simulink model "Seven_dof2017a"  (R2017a)
settings: Solver=ode45  StartTime=0.0  StopTime=10.0  RelTol=1e-3
values from neighbouring files (symbols this model uses):
  Bf = 1.6    [0108.mat]    (also in Sensor_wz_u1.m; Sensor_wz_u3.m; Sensor_wz_u4.m; unlinear_7DOF_Parameters.m)
  Br = 1.6    [0108.mat]    (also in Sensor_wz_u1.m; Sensor_wz_u3.m; Sensor_wz_u4.m; unlinear_7DOF_Parameters.m)
  f = 0.015    [0108.mat]    (also in unlinear_7DOF_Parameters.m)
  g = 9.8    [0108.mat]    (also in unlinear_7DOF_Parameters.m)
  hg = 0.5    [0108.mat]    (also in unlinear_7DOF_Parameters.m)
  i_sw = 20    [unlinear_7DOF_Parameters.m]
  I_tire = 2.5    [0108.mat]    (also in unlinear_7DOF_Parameters.m)
  Iz = 2700    [0108.mat]    (also in LinearState2_u.m = 1536.7; Sensor_wz_u1.m; Sensor_wz_u3.m; Sensor_wz_u4.m)
  L = 2.6    [0108.mat]    (also in unlinear_7DOF_Parameters.m)
  Lf = 1.2    [0108.mat]    (also in Sensor_wz_u1.m; Sensor_wz_u3.m; Sensor_wz_u4.m; unlinear_7DOF_Parameters.m)
  Lr = 1.4    [0108.mat]    (also in Sensor_wz_u1.m = 1.2; Sensor_wz_u3.m = 1.2; Sensor_wz_u4.m = 1.2; unlinear_7DOF_Parameters.m)
  m = 1765    [0108.mat]    (also in LinearState2_u.m = 1412; Sensor_ax_u0.m; Sensor_ax_u1.m; Sensor_ax_u2.m = 1412)
  mb = 1600    [0108.mat]    (also in unlinear_7DOF_Parameters.m)
  mw = 41.25    [0108.mat]    (also in unlinear_7DOF_Parameters.m)
  Pn_motor = 80    [unlinear_7DOF_Parameters.m]
  r = 0.324956275    [0108.mat]    (also in unlinear_7DOF_Parameters.m = 0.354)
  Tn_motor = 1000    [unlinear_7DOF_Parameters.m]
  u_fl = 0.3    [unlinear_7DOF_Parameters.m]
  u_fr = 0.8    [unlinear_7DOF_Parameters.m]
  u_rl = 0.3    [unlinear_7DOF_Parameters.m]
  u_rr = 0.8    [unlinear_7DOF_Parameters.m]
  v_obj = 16    [unlinear_7DOF_Parameters.m]
  vx0 = 16    [unlinear_7DOF_Parameters.m]
  w0 = vx0/r    (= 45.197740113)    [unlinear_7DOF_Parameters.m]
libraries: sharedTrackingLibrary x2, simulink x1
(part 1 of 2)
settings Model: Creator=dzY  LastModifiedBy=dzY
settings DataIOCC: LimitDataPoints=on  SaveFormat=Array
settings OptimizationCC: BlockReduction=off  BooleanDataType=off  LifeSpan=inf
settings DebuggingCC: SaveWithParameterizedLinksMsg=none  UnderspecifiedInitializationDetection=Classic  MergeDetectMultiDrivingBlocksExec=none  SignalResolutionControl=TryResolveAllWithWarning  SFUnexpectedBacktrackingDiag=warning  SFNoUnconditionalDefaultTransitionDiag=warning  SFExecutionAtInitializationDiag=none
settings HardwareCC: ProdBitPerPointer=32  ProdBitPerSizeT=32  ProdBitPerPtrDiffT=32  ProdLargestAtomicFloat=None  ProdIntDivRoundTo=Undefined  ProdEndianess=Unspecified  ProdWordSize=32  ProdHWDeviceType=32-bit Generic  TargetUnknown=on
settings ModelReferenceCC: PropagateSignalLabelsOutOfModel=off
settings GRTTargetCC: TargetLangStandard=C89/C90 (ANSI)  GeneratePreprocessorConditionals=Disable all
settings ConfigComp: CovMetricSettings=dw  CovHtmlReporting=on  CovSaveCumulativeToWorkspaceVar=on  CovSaveSingleToWorkspaceVar=on  CovExternalEMLEnable=off  CovSFcnEnable=off

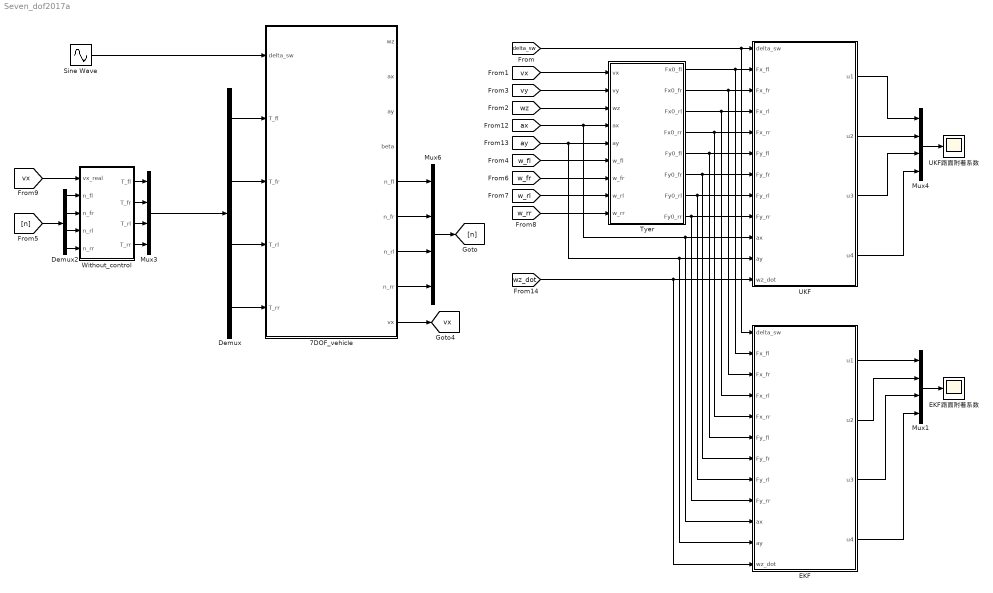
== system Seven_dof2017a ==
  7DOF_vehicle : Subsystem
  Demux : Demux
  Demux2 : Demux
  EKF : Subsystem
  EKF路面附着系数 : Scope
  Mux{1,3..4,6} (4 alike) : Mux
  Sine Wave : Sin  Amplitude=0.1  SampleTime=0
  Tyer : Subsystem
  UKF : Subsystem
  UKF路面附着系数 : Scope
  Without_control : Subsystem
  tag scope: vx=global
  wires:
  Without_control/1(T_fl) -> Mux3/1
  Without_control/2(T_fr) -> Mux3/2
  Without_control/3(T_rl) -> Mux3/3
  Without_control/4(T_rr) -> Mux3/4
  Demux2/1 -> Without_control/2(n_fl)
  Demux2/2 -> Without_control/3(n_fr)
  Demux2/4 -> Without_control/5(n_rr)
  Demux2/3 -> Without_control/4(n_rl)
  [n] -> Demux2/1
  [vx] -> Without_control/1(vx_real)
  7DOF_vehicle/9(vx) -> [vx]
  Mux6/1 -> [n]
  7DOF_vehicle/5(n_fl) -> Mux6/1
  7DOF_vehicle/6(n_fr) -> Mux6/2
  7DOF_vehicle/7(n_rl) -> Mux6/3
  7DOF_vehicle/8(n_rr) -> Mux6/4
  Demux/1 -> 7DOF_vehicle/2(T_fl)
  Demux/2 -> 7DOF_vehicle/3(T_fr)
  Demux/3 -> 7DOF_vehicle/4(T_rl)
  Demux/4 -> 7DOF_vehicle/5(T_rr)
  Mux3/1 -> Demux/1
  UKF/2(u2) -> Mux4/2
  UKF/1(u1) -> Mux4/1
  Mux4/1 -> UKF路面附着系数/1
  UKF/4(u4) -> Mux4/4
  UKF/3(u3) -> Mux4/3
  Tyer/1(Fx0_fl) -> EKF/2(Fx_fl), UKF/2(Fx_fl)
  Tyer/2(Fx0_fr) -> EKF/3(Fx_fr), UKF/3(Fx_fr)
  Tyer/3(Fx0_rl) -> EKF/4(Fx_rl), UKF/4(Fx_rl)
  Tyer/4(Fx0_rr) -> EKF/5(Fx_rr), UKF/5(Fx_rr)
  Tyer/5(Fy0_fl) -> EKF/6(Fy_fl), UKF/6(Fy_fl)
  Tyer/6(Fy0_fr) -> EKF/7(Fy_fr), UKF/7(Fy_fr)
  Tyer/7(Fy0_rl) -> EKF/8(Fy_rl), UKF/8(Fy_rl)
  Tyer/8(Fy0_rr) -> EKF/9(Fy_rr), UKF/9(Fy_rr)
  [delta_sw] -> EKF/1(delta_sw), UKF/1(delta_sw)
  [ay] -> EKF/11(ay), UKF/11(ay), Tyer/5(ay)
  [vx] -> Tyer/1(vx)
  [wz] -> Tyer/3(wz)
  [vy] -> Tyer/2(vy)
  [wz_dot] -> EKF/12(wz_dot), UKF/12(wz_dot)
  [w_fl] -> Tyer/6(w_fl)
  [w_fr] -> Tyer/7(w_fr)
  [w_rl] -> Tyer/8(w_rl)
  [w_rr] -> Tyer/9(w_rr)
  [ax] -> EKF/10(ax), UKF/10(ax), Tyer/4(ax)
  Sine Wave/1 -> 7DOF_vehicle/1(delta_sw)
  EKF/1(u1) -> Mux1/1
  EKF/2(u2) -> Mux1/2
  EKF/4(u4) -> Mux1/4
  EKF/3(u3) -> Mux1/3
  Mux1/1 -> EKF路面附着系数/1

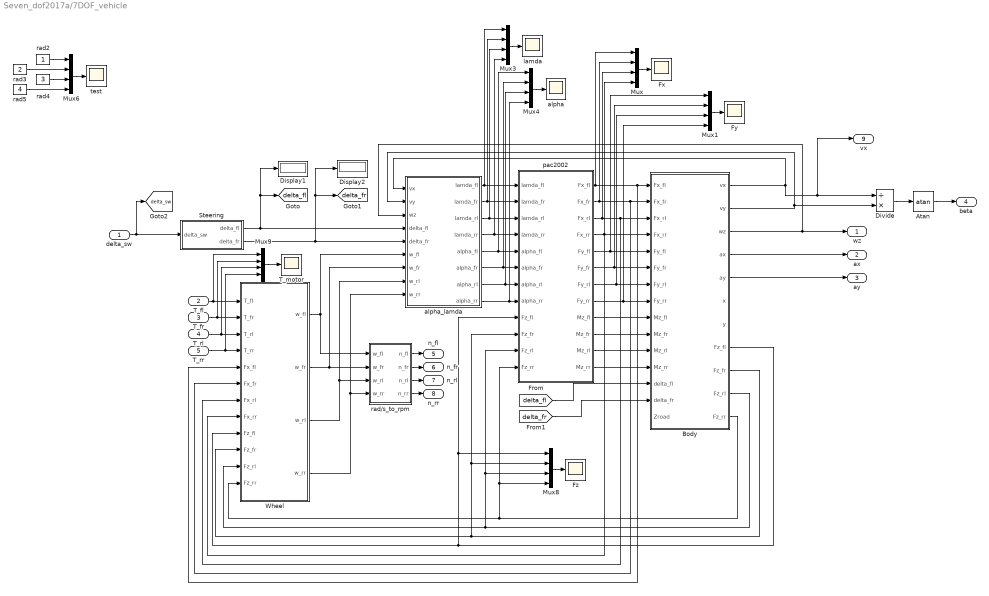
== system Seven_dof2017a/7DOF_vehicle ==
  delta_sw : Inport
  T_fl : Inport  Port=2
  T_fr : Inport  Port=3
  T_rl : Inport  Port=4
  T_rr : Inport  Port=5
  Atan : Trigonometry  Operator=atan
  Body : Subsystem
  Display1 : Display
  Display2 : Display
  Divide : Product  Inputs=/*
  Fx : Scope
  Fy : Scope
  Fz : Scope
  Mux{,1,3..4,6,8..9} (7 alike) : Mux
  Steering : Subsystem
  T_motor : Scope
  Wheel : Subsystem
  alpha : Scope
  alpha_lamda : Subsystem
  lamda : Scope
  pac2002 : Subsystem
  rad/s_to_rpm : Subsystem
  rad2 : Constant
  rad3 : Constant  Value=2
  rad4 : Constant  Value=3
  rad5 : Constant  Value=4
  test : Scope
  wz : Outport
  ax : Outport  Port=2
  ay : Outport  Port=3
  beta : Outport  Port=4
  n_fl : Outport  Port=5
  n_fr : Outport  Port=6
  n_rl : Outport  Port=7
  n_rr : Outport  Port=8
  vx : Outport  Port=9
  tag scope: delta_fl=global, delta_fr=global, delta_sw=global
  wires:
  pac2002/12(Mz_rr) -> Body/12(Mz_rr)
  pac2002/11(Mz_rl) -> Body/11(Mz_rl)
  pac2002/10(Mz_fr) -> Body/10(Mz_fr)
  pac2002/9(Mz_fl) -> Body/9(Mz_fl)
  Atan/1 -> beta/1
  Divide/1 -> Atan/1
  T_rr/1 -> Wheel/4(T_rr), Mux9/4
  rad/s_to_rpm/4(n_rr) -> n_rr/1
  rad/s_to_rpm/2(n_fr) -> n_fr/1
  T_rl/1 -> Wheel/3(T_rl), Mux9/3
  Body/5(ay) -> ay/1
  Body/1(vx) -> vx/1, Divide/1, alpha_lamda/1(vx)
  Mux6/1 -> test/1
  Wheel/4(w_rr) -> rad/s_to_rpm/4(w_rr), alpha_lamda/9(w_rr)
  rad3/1 -> Mux6/2
  delta_sw/1 -> [delta_sw], Steering/1(delta_sw)
  Body/2(vy) -> alpha_lamda/2(vy), Divide/2
  rad4/1 -> Mux6/3
  rad5/1 -> Mux6/4
  Mux3/1 -> lamda/1
  Mux/1 -> Fx/1
  T_fl/1 -> Wheel/1(T_fl), Mux9/1
  Body/11(Fz_rr) -> pac2002/12(Fz_rr), Mux8/4, Wheel/12(Fz_rr)
  Mux4/1 -> alpha/1
  rad/s_to_rpm/3(n_rl) -> n_rl/1
  T_fr/1 -> Wheel/2(T_fr), Mux9/2
  pac2002/3(Fx_rl) -> Wheel/7(Fx_rl), Body/3(Fx_rl), Mux/3
  alpha_lamda/6(alpha_fr) -> pac2002/6(alpha_fr), Mux4/2
  Body/9(Fz_fr) -> pac2002/10(Fz_fr), Mux8/2, Wheel/10(Fz_fr)
  [delta_fr] -> Body/14(delta_fr)
  alpha_lamda/5(alpha_fl) -> pac2002/5(alpha_fl), Mux4/1
  alpha_lamda/8(alpha_rr) -> pac2002/8(alpha_rr), Mux4/4
  Wheel/1(w_fl) -> rad/s_to_rpm/1(w_fl), alpha_lamda/6(w_fl)
  Wheel/3(w_rl) -> rad/s_to_rpm/3(w_rl), alpha_lamda/8(w_rl)
  Body/10(Fz_rl) -> pac2002/11(Fz_rl), Mux8/3, Wheel/11(Fz_rl)
  Mux9/1 -> T_motor/1
  Mux1/1 -> Fy/1
  rad/s_to_rpm/1(n_fl) -> n_fl/1
  alpha_lamda/7(alpha_rl) -> pac2002/7(alpha_rl), Mux4/3
  Mux8/1 -> Fz/1
  Wheel/2(w_fr) -> rad/s_to_rpm/2(w_fr), alpha_lamda/7(w_fr)
  pac2002/8(Fy_rr) -> Body/8(Fy_rr), Mux1/4
  alpha_lamda/2(lamda_fr) -> pac2002/2(lamda_fr), Mux3/2
  pac2002/5(Fy_fl) -> Mux1/1, Body/5(Fy_fl)
  pac2002/2(Fx_fr) -> Wheel/6(Fx_fr), Body/2(Fx_fr), Mux/2
  Body/8(Fz_fl) -> pac2002/9(Fz_fl), Mux8/1, Wheel/9(Fz_fl)
  alpha_lamda/3(lamda_rl) -> pac2002/3(lamda_rl), Mux3/3
  pac2002/6(Fy_fr) -> Body/6(Fy_fr), Mux1/2
  pac2002/7(Fy_rl) -> Body/7(Fy_rl), Mux1/3
  Steering/2(delta_fr) -> alpha_lamda/5(delta_fr), Display2/1, [delta_fr]
  Steering/1(delta_fl) -> alpha_lamda/4(delta_fl), Display1/1, [delta_fl]
  alpha_lamda/4(lamda_rr) -> pac2002/4(lamda_rr), Mux3/4
  alpha_lamda/1(lamda_fl) -> pac2002/1(lamda_fl), Mux3/1
  pac2002/1(Fx_fl) -> Wheel/5(Fx_fl), Body/1(Fx_fl), Mux/1
  rad2/1 -> Mux6/1
  [delta_fl] -> Body/13(delta_fl)
  Body/3(wz) -> wz/1, alpha_lamda/3(wz)
  pac2002/4(Fx_rr) -> Mux/4, Wheel/8(Fx_rr), Body/4(Fx_rr)
  Body/4(ax) -> ax/1

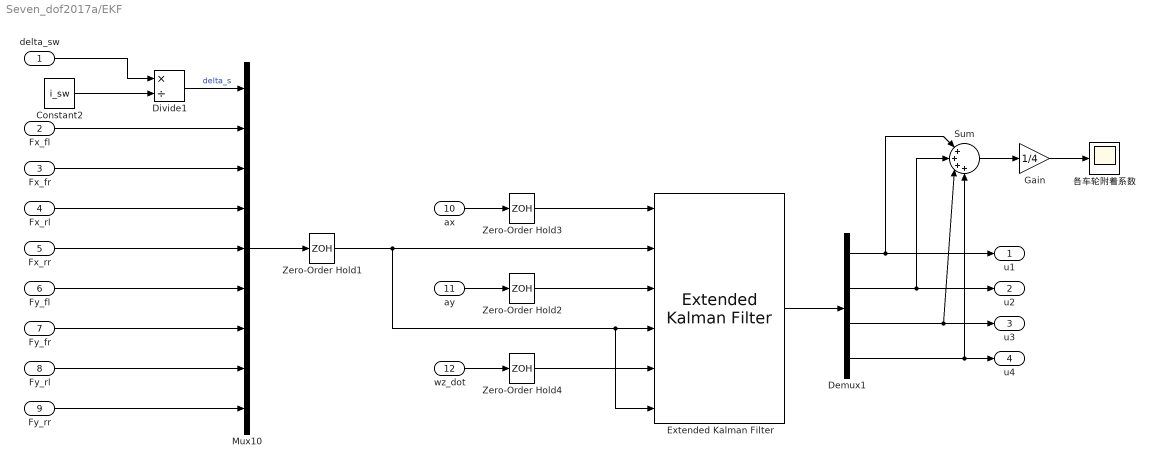
== system Seven_dof2017a/EKF ==
  delta_sw : Inport
  Fx_fl : Inport  Port=2
  Fx_fr : Inport  Port=3
  Fx_rl : Inport  Port=4
  Fx_rr : Inport  Port=5
  Fy_fl : Inport  Port=6
  Fy_fr : Inport  Port=7
  Fy_rl : Inport  Port=8
  Fy_rr : Inport  Port=9
  ax : Inport  Port=10
  ay : Inport  Port=11
  wz_dot : Inport  Port=12
  Constant2 : Constant  Value=i_sw
  Demux1 : Demux
  Divide1 : Product  Inputs=*/
  Extended Kalman Filter : sharedTrackingLibrary/Extended Kalman Filter  StateTransitionFcn=LinearState_u  HasStateTransitionJacobianFcn=off  HasAdditiveProcessNoise=Additive  ProcessNoise=diag([0.1 0.1 0.1 0.1])  HasTimeVaryingProcessNoise=off  HasStateTransitionFcnExtraArgument=0  InitialState=[1;1; 1; 1]  InitialStateCovariance=1e-4  MeasurementFcn1=Sensor_ax_u  HasMeasurementJacobianFcn1=off  HasMeasurementEnablePort1=off  HasAdditiveMeasurementNoise1=Additive  MeasurementNoise1=0.0001  HasTimeVaryingMeasurementNoise1=off  HasMeasurementFcnExtraArgument1=1  MeasurementFcn2=Sensor_ay_u  HasMeasurementJacobianFcn2=off  HasMeasurementEnablePort2=off  HasAdditiveMeasurementNoise2=Additive  MeasurementNoise2=0.0001  HasTimeVaryingMeasurementNoise2=off  HasMeasurementFcnExtraArgument2=1  MeasurementFcn3=Sensor_wz_u  HasMeasurementJacobianFcn3=off  HasMeasurementEnablePort3=off  HasAdditiveMeasurementNoise3=Additive  MeasurementNoise3=0.0001  HasTimeVaryingMeasurementNoise3=off  HasMeasurementFcnExtraArgument3=1  MeasurementFcn4=myMeasurementFcn  HasMeasurementJacobianFcn4=off  HasMeasurementEnablePort4=off  HasAdditiveMeasurementNoise4=Additive  MeasurementNoise4=1  HasTimeVaryingMeasurementNoise4=off  HasMeasurementFcnExtraArgument4=0  MeasurementFcn5=myMeasurementFcn  HasMeasurementJacobianFcn5=off  HasMeasurementEnablePort5=off  HasAdditiveMeasurementNoise5=Additive  MeasurementNoise5=1  HasTimeVaryingMeasurementNoise5=off  HasMeasurementFcnExtraArgument5=0  EnableMultirate=on  StateTransitionFcnSampleTime=0.01  MeasurementFcn1SampleTime=0.01  MeasurementFcn2SampleTime=0.01  MeasurementFcn3SampleTime=0.01  MeasurementFcn4SampleTime=1  MeasurementFcn5SampleTime=1  UseCurrentEstimator=on  OutputStateCovariance=off  DataType=double  SampleTime=0.01  NumberOfMeasurements=3
      settings: SourceProductName=Control System Toolbox  SourceProductBaseCode=CT
  Gain : Gain  Gain=1/4
  Mux10 : Mux  Inputs=9
  Sum : Sum  Inputs=|++++
  Zero-Order Hold{1..4} (4 alike) : ZeroOrderHold  SampleTime=0.01
  各车轮附着系数 : Scope
  u1 : Outport
  u2 : Outport  Port=2
  u3 : Outport  Port=3
  u4 : Outport  Port=4
  wires:
  Gain/1 -> 各车轮附着系数/1
  Sum/1 -> Gain/1
  Zero-Order Hold3/1 -> Extended Kalman Filter/1
  Zero-Order Hold2/1 -> Extended Kalman Filter/3
  Demux1/4 -> Sum/4, u4/1
  Zero-Order Hold1/1 -> Extended Kalman Filter/2, Extended Kalman Filter/6, Extended Kalman Filter/4
  Fy_rr/1 -> Mux10/9
  Fy_rl/1 -> Mux10/8
  Fy_fr/1 -> Mux10/7
  Fy_fl/1 -> Mux10/6
  Fx_rr/1 -> Mux10/5
  Fx_rl/1 -> Mux10/4
  Fx_fr/1 -> Mux10/3
  Fx_fl/1 -> Mux10/2
  Zero-Order Hold4/1 -> Extended Kalman Filter/5
  wz_dot/1 -> Zero-Order Hold4/1
  ay/1 -> Zero-Order Hold2/1
  ax/1 -> Zero-Order Hold3/1
  Constant2/1 -> Divide1/2
  delta_sw/1 -> Divide1/1
  Extended Kalman Filter/1 -> Demux1/1
  Mux10/1 -> Zero-Order Hold1/1
  Divide1/1 -> Mux10/1  "delta_s"
  Demux1/1 -> u1/1, Sum/1
  Demux1/3 -> Sum/3, u3/1
  Demux1/2 -> u2/1, Sum/2

== system Seven_dof2017a/Tyer ==
  vx : Inport
  vy : Inport  Port=2
  wz : Inport  Port=3
  ax : Inport  Port=4
  ay : Inport  Port=5
  w_fl : Inport  Port=6
  w_fr : Inport  Port=7
  w_rl : Inport  Port=8
  w_rr : Inport  Port=9
  Fz : Subsystem
  alpha_lamda : Subsystem
  pac2002 : Subsystem
  Fx0_fl : Outport
  Fx0_fr : Outport  Port=2
  Fx0_rl : Outport  Port=3
  Fx0_rr : Outport  Port=4
  Fy0_fl : Outport  Port=5
  Fy0_fr : Outport  Port=6
  Fy0_rl : Outport  Port=7
  Fy0_rr : Outport  Port=8
  wires:
  ay/1 -> Fz/2(ay)
  ax/1 -> Fz/1(ax)
  [delta_s] -> alpha_lamda/5(delta_fr), alpha_lamda/4(delta_fl)
  vx/1 -> alpha_lamda/1(vx)
  vy/1 -> alpha_lamda/2(vy)
  wz/1 -> alpha_lamda/3(wz)
  w_fl/1 -> alpha_lamda/6(w_fl)
  w_fr/1 -> alpha_lamda/7(w_fr)
  w_rl/1 -> alpha_lamda/8(w_rl)
  w_rr/1 -> alpha_lamda/9(w_rr)
  alpha_lamda/1(lamda_fl) -> pac2002/1(lamda_fl)
  alpha_lamda/2(lamda_fr) -> pac2002/2(lamda_fr)
  alpha_lamda/3(lamda_rl) -> pac2002/3(lamda_rl)
  alpha_lamda/4(lamda_rr) -> pac2002/4(lamda_rr)
  alpha_lamda/5(alpha_fl) -> pac2002/5(alpha_fl)
  alpha_lamda/6(alpha_fr) -> pac2002/6(alpha_fr)
  alpha_lamda/7(alpha_rl) -> pac2002/7(alpha_rl)
  alpha_lamda/8(alpha_rr) -> pac2002/8(alpha_rr)
  Fz/1(Fz_fl) -> pac2002/9(Fz_fl)
  Fz/2(Fz_fr) -> pac2002/10(Fz_fr)
  Fz/3(Fz_rl) -> pac2002/11(Fz_rl)
  Fz/4(Fz_rr) -> pac2002/12(Fz_rr)
  pac2002/1(Fx0_fl) -> Fx0_fl/1
  pac2002/2(Fx0_fr) -> Fx0_fr/1
  pac2002/3(Fx0_rl) -> Fx0_rl/1
  pac2002/4(Fx0_rr) -> Fx0_rr/1
  pac2002/5(Fy0_fl) -> Fy0_fl/1
  pac2002/6(Fy0_fr) -> Fy0_fr/1
  pac2002/7(Fy0_rl) -> Fy0_rl/1
  pac2002/8(Fy_rr) -> Fy0_rr/1

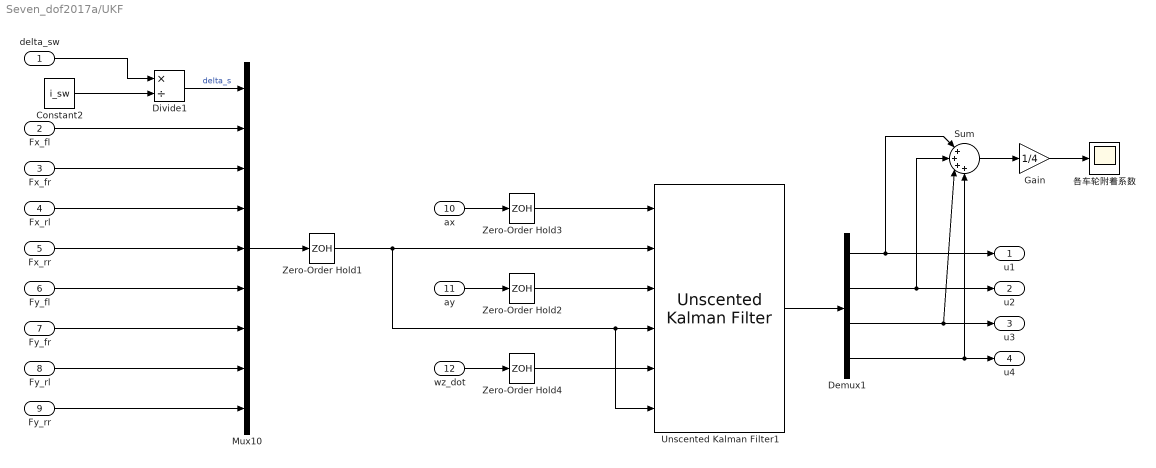
== system Seven_dof2017a/UKF ==
  delta_sw : Inport
  Fx_fl : Inport  Port=2
  Fx_fr : Inport  Port=3
  Fx_rl : Inport  Port=4
  Fx_rr : Inport  Port=5
  Fy_fl : Inport  Port=6
  Fy_fr : Inport  Port=7
  Fy_rl : Inport  Port=8
  Fy_rr : Inport  Port=9
  ax : Inport  Port=10
  ay : Inport  Port=11
  wz_dot : Inport  Port=12
  Constant2 : Constant  Value=i_sw
  Demux1 : Demux
  Divide1 : Product  Inputs=*/
  Gain : Gain  Gain=1/4
  Mux10 : Mux  Inputs=9
  Sum : Sum  Inputs=|++++
  Unscented Kalman Filter1 : sharedTrackingLibrary/Unscented Kalman Filter  StateTransitionFcn=LinearState_u  HasAdditiveProcessNoise=Additive  ProcessNoise=diag([0.1 0.1 0.1 0.1])  HasTimeVaryingProcessNoise=off  HasStateTransitionFcnExtraArgument=0  InitialState=[1;1; 1; 1]  InitialStateCovariance=1e-4  Alpha=1e-3  Beta=2  Kappa=0  MeasurementFcn1=Sensor_ax_u  HasMeasurementEnablePort1=off  HasAdditiveMeasurementNoise1=Additive  MeasurementNoise1=0.0001  HasTimeVaryingMeasurementNoise1=off  HasMeasurementFcnExtraArgument1=1  MeasurementFcn2=Sensor_ay_u  HasMeasurementEnablePort2=off  HasAdditiveMeasurementNoise2=Additive  MeasurementNoise2=0.0001  HasTimeVaryingMeasurementNoise2=off  HasMeasurementFcnExtraArgument2=1  MeasurementFcn3=Sensor_wz_u  HasMeasurementEnablePort3=off  HasAdditiveMeasurementNoise3=Additive  MeasurementNoise3=0.0001  HasTimeVaryingMeasurementNoise3=off  HasMeasurementFcnExtraArgument3=1  MeasurementFcn4=myMeasurementFcn  HasMeasurementEnablePort4=off  HasAdditiveMeasurementNoise4=Additive  MeasurementNoise4=1  HasTimeVaryingMeasurementNoise4=off  HasMeasurementFcnExtraArgument4=0  MeasurementFcn5=myMeasurementFcn  HasMeasurementEnablePort5=off  HasAdditiveMeasurementNoise5=Additive  MeasurementNoise5=1  HasTimeVaryingMeasurementNoise5=off  HasMeasurementFcnExtraArgument5=0  EnableMultirate=on  StateTransitionFcnSampleTime=0.01  MeasurementFcn1SampleTime=0.01  MeasurementFcn2SampleTime=0.01  MeasurementFcn3SampleTime=0.01  MeasurementFcn4SampleTime=1  MeasurementFcn5SampleTime=1  UseCurrentEstimator=on  OutputStateCovariance=off  DataType=double  SampleTime=1  NumberOfMeasurements=3
      settings: SourceProductName=Control System Toolbox  SourceProductBaseCode=CT
  Zero-Order Hold{1..4} (4 alike) : ZeroOrderHold  SampleTime=0.01
  各车轮附着系数 : Scope
  u1 : Outport
  u2 : Outport  Port=2
  u3 : Outport  Port=3
  u4 : Outport  Port=4
  wires:
  Demux1/2 -> Sum/2, u2/1
  Demux1/3 -> u3/1, Sum/3
  Demux1/1 -> Sum/1, u1/1
  Divide1/1 -> Mux10/1  "delta_s"
  Mux10/1 -> Zero-Order Hold1/1
  Unscented Kalman Filter1/1 -> Demux1/1
  delta_sw/1 -> Divide1/1
  Constant2/1 -> Divide1/2
  ax/1 -> Zero-Order Hold3/1
  ay/1 -> Zero-Order Hold2/1
  wz_dot/1 -> Zero-Order Hold4/1
  Zero-Order Hold4/1 -> Unscented Kalman Filter1/5
  Fx_fl/1 -> Mux10/2
  Fx_fr/1 -> Mux10/3
  Fx_rl/1 -> Mux10/4
  Fx_rr/1 -> Mux10/5
  Fy_fl/1 -> Mux10/6
  Fy_fr/1 -> Mux10/7
  Fy_rl/1 -> Mux10/8
  Fy_rr/1 -> Mux10/9
  Zero-Order Hold1/1 -> Unscented Kalman Filter1/2, Unscented Kalman Filter1/6, Unscented Kalman Filter1/4
  Demux1/4 -> u4/1, Sum/4
  Zero-Order Hold2/1 -> Unscented Kalman Filter1/3
  Zero-Order Hold3/1 -> Unscented Kalman Filter1/1
  Sum/1 -> Gain/1
  Gain/1 -> 各车轮附着系数/1

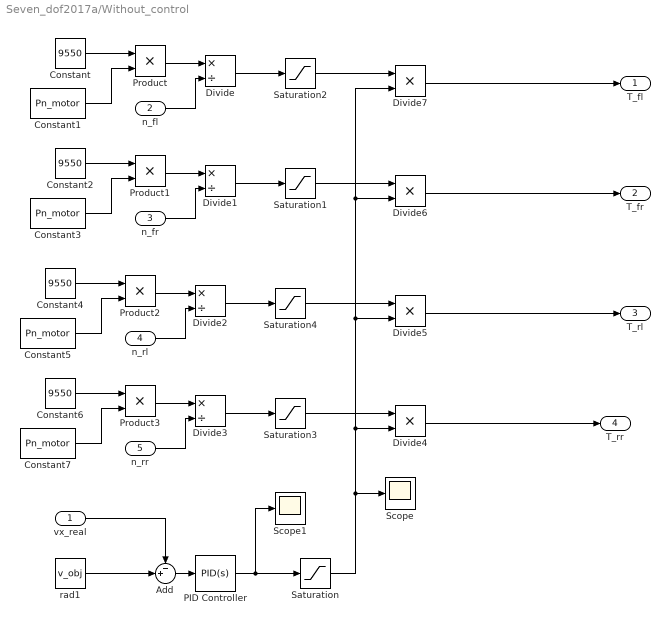
== system Seven_dof2017a/Without_control ==
  vx_real : Inport
  n_fl : Inport  Port=2
  n_fr : Inport  Port=3
  n_rl : Inport  Port=4
  n_rr : Inport  Port=5
  Add : Sum  Inputs=-+|
  Constant{,2,4,6} (4 alike) : Constant  Value=9550
  Constant{1,3,5,7} (4 alike) : Constant  Value=Pn_motor
  Divide{,1..3} (4 alike) : Product  Inputs=*/
  Divide{4..7} (4 alike) : Product  Inputs=**
  PID Controller : simulink/Continuous/PID Controller  Controller=PID  Form=Parallel  TimeDomain=Continuous-time  SampleTime=-1  IntegratorMethod=Forward Euler  FilterMethod=Forward Euler  ControllerParametersSource=internal  P=1  I=1  D=0  UseFilter=on  N=100  InitialConditionSource=internal  InitialConditionForIntegrator=0  InitialConditionForFilter=0  DifferentiatorICPrevScaledInput=0  ExternalReset=none  TrackingMode=off  Kt=1  LimitOutput=off  UpperSaturationLimit=inf  LowerSaturationLimit=-inf  LinearizeAsGain=on  AntiWindupMode=none  Kb=1  POutMin=[]  POutMax=[]  IOutMin=[]  IOutMax=[]  DOutMin=[]  DOutMax=[]  NOutMin=[]  NOutMax=[]  SumOutMin=[]  SumOutMax=[]  SaturationOutMin=[]  SaturationOutMax=[]  PParamMin=[]  PParamMax=[]  IParamMin=[]  IParamMax=[]  DParamMin=[]  DParamMax=[]  NParamMin=[]  NParamMax=[]  KbParamMin=[]  KbParamMax=[]  KtParamMin=[]  KtParamMax=[]  KbOutMin=[]  KbOutMax=[]  KtOutMin=[]  KtOutMax=[]  IntegratorOutMin=[]  IntegratorOutMax=[]  FilterOutMin=[]  FilterOutMax=[]  SumI1OutMin=[]  SumI1OutMax=[]  SumI2OutMin=[]  SumI2OutMax=[]  SumI3OutMin=[]  SumI3OutMax=[]  SumDOutMin=[]  SumDOutMax=[]  DifferentiatorOutMin=[]  DifferentiatorOutMax=[]  IntegratorContinuousStateAttributes=''  IntegratorStateMustResolveToSignalObject=off  IntegratorRTWStateStorageClass=Auto  FilterContinuousStateAttributes=''  FilterStateMustResolveToSignalObject=off  FilterRTWStateStorageClass=Auto
  Product{,1..3} (4 alike) : Product
  Saturation : Saturate  UpperLimit=1  LowerLimit=-1
  Saturation{1..4} (4 alike) : Saturate  UpperLimit=Tn_motor  LowerLimit=-Tn_motor
  Scope : Scope
  Scope1 : Scope
  rad1 : Constant  Value=v_obj
  T_fl : Outport
  T_fr : Outport  Port=2
  T_rl : Outport  Port=3
  T_rr : Outport  Port=4
  wires:
  Saturation/1 -> Divide7/2, Divide6/2, Divide5/2, Divide4/2, Scope/1
  Add/1 -> PID Controller/1
  rad1/1 -> Add/2
  PID Controller/1 -> Saturation/1, Scope1/1
  Divide4/1 -> T_rr/1
  Divide5/1 -> T_rl/1
  Divide6/1 -> T_fr/1
  Divide7/1 -> T_fl/1
  vx_real/1 -> Add/1
  n_fl/1 -> Divide/2
  Divide/1 -> Saturation2/1
  Constant/1 -> Product/1
  Constant1/1 -> Product/2
  Product/1 -> Divide/1
  n_fr/1 -> Divide1/2
  Divide1/1 -> Saturation1/1
  Constant2/1 -> Product1/1
  Constant3/1 -> Product1/2
  Product1/1 -> Divide1/1
  n_rl/1 -> Divide2/2
  Divide2/1 -> Saturation4/1
  Constant4/1 -> Product2/1
  Constant5/1 -> Product2/2
  Product2/1 -> Divide2/1
  n_rr/1 -> Divide3/2
  Divide3/1 -> Saturation3/1
  Constant6/1 -> Product3/1
  Constant7/1 -> Product3/2
  Product3/1 -> Divide3/1
  Saturation3/1 -> Divide4/1
  Saturation4/1 -> Divide5/1
  Saturation1/1 -> Divide6/1
  Saturation2/1 -> Divide7/1

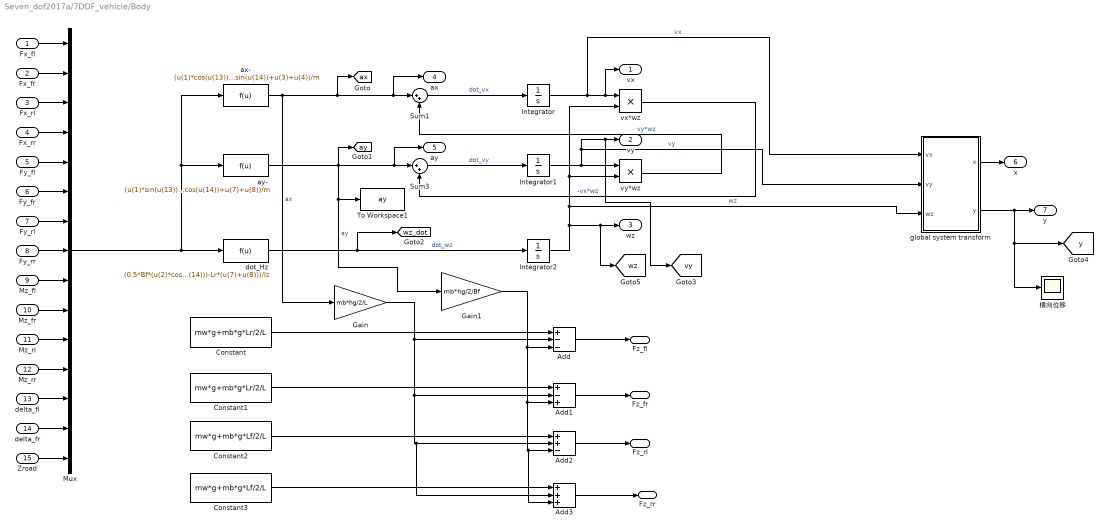
== system Seven_dof2017a/7DOF_vehicle/Body ==
  Fx_fl : Inport
  Fx_fr : Inport  Port=2
  Fx_rl : Inport  Port=3
  Fx_rr : Inport  Port=4
  Fy_fl : Inport  Port=5
  Fy_fr : Inport  Port=6
  Fy_rl : Inport  Port=7
  Fy_rr : Inport  Port=8
  Mz_fl : Inport  Port=9
  Mz_fr : Inport  Port=10
  Mz_rl : Inport  Port=11
  Mz_rr : Inport  Port=12
  delta_fl : Inport  Port=13
  delta_fr : Inport  Port=14
  Zroad : Inport  Port=15
  Add : Sum  Inputs=+--
  Add1 : Sum  Inputs=+-+
  Add2 : Sum  Inputs=++-
  Add3 : Sum  Inputs=+++
  Constant : Constant  Value=mw*g+mb*g*Lr/2/L
  Constant1 : Constant  Value=mw*g+mb*g*Lr/2/L
  Constant2 : Constant  Value=mw*g+mb*g*Lf/2/L
  Constant3 : Constant  Value=mw*g+mb*g*Lf/2/L
  Gain : Gain  Gain=mb*hg/2/L
  Gain1 : Gain  Gain=mb*hg/2/Bf
  Integrator : Integrator  InitialCondition=vx0  LimitOutput=on  LowerSaturationLimit=0
  Integrator1 : Integrator
  Integrator2 : Integrator
  Mux : Mux  Inputs=15
  Sum1 : Sum  Inputs=|++
  Sum3 : Sum  Inputs=|++
  To Workspace1 : ToWorkspace  VariableName=ay  SaveFormat=Timeseries  SampleTime=-1
  ax- : Fcn  Expr=(u(1)*cos(u(13))+u(2)*cos(u(14))-u(5)*sin(u(13))-u(6)*sin(u(14))+u(3)+u(4))/m
  ay- : Fcn  Expr=(u(1)*sin(u(13))+u(2)*sin(u(14))+u(5)*cos(u(13))+u(6)*cos(u(14))+u(7)+u(8))/m
  dot_Hz : Fcn  Expr=(0.5*Bf*(u(2)*cos(u(14))-u(1)*cos(u(13))-u(6)*sin(u(14))+u(5)*sin(u(13)))+0.5*Br*(u(4)-u(3))+Lf*(u(1)*sin(u(13))+u(5)*cos(u(13))+u(2)*sin(u(14))+u(6)*cos(u(14)))-Lr*(u(7)+u(8)))/Iz
  global system transform : Subsystem
  vx*wz : Product
  vy*wz : Product
  横向位移 : Scope
  vx : Outport
  vy : Outport  Port=2
  wz : Outport  Port=3
  ax : Outport  Port=4
  ay : Outport  Port=5
  x : Outport  Port=6
  y : Outport  Port=7
  Fz_fl : Outport  Port=8
  Fz_fr : Outport  Port=9
  Fz_rl : Outport  Port=10
  Fz_rr : Outport  Port=11
  tag scope: ax=global, ay=global, vy=global, wz=global, wz_dot=global, y=global
  wires:
  global system transform/2(y) -> y/1, 横向位移/1, [y]
  global system transform/1(x) -> x/1
  Zroad/1 -> Mux/15
  Mux/1 -> dot_Hz/1, ay-/1, ax-/1
  delta_fr/1 -> Mux/14
  delta_fl/1 -> Mux/13
  Mz_rr/1 -> Mux/12
  Mz_rl/1 -> Mux/11
  Mz_fr/1 -> Mux/10
  Mz_fl/1 -> Mux/9
  Fy_rr/1 -> Mux/8
  Fy_rl/1 -> Mux/7
  Fy_fr/1 -> Mux/6
  Fy_fl/1 -> Mux/5
  Fx_rr/1 -> Mux/4
  Fx_rl/1 -> Mux/3
  Fx_fr/1 -> Mux/2
  Fx_fl/1 -> Mux/1
  Sum1/1 -> Integrator/1  "dot_vx"
  Integrator/1 -> vx/1, vx*wz/1, global system transform/1(vx)  "vx"
  Integrator1/1 -> global system transform/2(vy), [vy], vy/1, vy*wz/1  "vy"
  Sum3/1 -> Integrator1/1  "dot_vy"
  dot_Hz/1 -> Integrator2/1, [wz_dot]  "dot_wz"
  Integrator2/1 -> global system transform/3(wz), vy*wz/2, vx*wz/2, [wz], wz/1  "wz"
  ay-/1 -> Gain1/1, To Workspace1/1, ay/1, Sum3/1, [ay]  "ay"
  vy*wz/1 -> Sum1/2  "vy*wz"
  vx*wz/1 -> Sum3/2  "-vx*wz"
  ax-/1 -> Gain/1, ax/1, Sum1/1, [ax]  "ax"
  Constant/1 -> Add/1
  Gain/1 -> Add3/2, Add2/2, Add1/2, Add/2
  Gain1/1 -> Add3/3, Add2/3, Add1/3, Add/3
  Add/1 -> Fz_fl/1
  Constant1/1 -> Add1/1
  Add1/1 -> Fz_fr/1
  Constant2/1 -> Add2/1
  Add2/1 -> Fz_rl/1
  Constant3/1 -> Add3/1
  Add3/1 -> Fz_rr/1

== system Seven_dof2017a/7DOF_vehicle/Steering ==
  delta_sw : Inport
  Add : Sum
  Add2 : Sum  Inputs=-+
  Add3 : Sum
  Constant : Constant  Value=Lr
  Constant1 : Constant  Value=Lf
  Constant2 : Constant  Value=i_sw
  Constant3 : Constant  Value=Br
  Divide : Product  Inputs=*/
  Divide1 : Product  Inputs=/*
  Divide2 : Product  Inputs=/*
  Gain : Gain  Gain=2
  Gain1 : Gain  Gain=57
  Product : Product
  Product1 : Product
  Trigonometric Function : Trigonometry  Operator=atan
  Trigonometric Function1 : Trigonometry  Operator=tan
  Trigonometric Function2 : Trigonometry  Operator=atan
  前轮转角 : Scope
  delta_fl : Outport
  delta_fr : Outport  Port=2
  tag scope: delta_s=global
  wires:
  Trigonometric Function2/1 -> delta_fr/1
  Divide2/1 -> Trigonometric Function2/1
  Add3/1 -> Divide2/1
  Trigonometric Function/1 -> delta_fl/1
  Divide1/1 -> Trigonometric Function/1
  Product/1 -> Divide1/2, Divide2/2
  Add2/1 -> Divide1/1
  Product1/1 -> Add2/1, Add3/1
  Constant3/1 -> Product1/1
  Gain/1 -> Add2/2, Add3/2, Product/2
  Trigonometric Function1/1 -> Product1/2, Product/1
  Divide/1 -> Trigonometric Function1/1, Gain1/1, [delta_s]  "delta_s"
  Constant2/1 -> Divide/2
  delta_sw/1 -> Divide/1
  Add/1 -> Gain/1
  Constant/1 -> Add/2
  Constant1/1 -> Add/1
  Gain1/1 -> 前轮转角/1

== system Seven_dof2017a/7DOF_vehicle/Wheel ==
  T_fl : Inport
  T_fr : Inport  Port=2
  T_rl : Inport  Port=3
  T_rr : Inport  Port=4
  Fx_fl : Inport  Port=5
  Fx_fr : Inport  Port=6
  Fx_rl : Inport  Port=7
  Fx_rr : Inport  Port=8
  Fz_fl : Inport  Port=9
  Fz_fr : Inport  Port=10
  Fz_rl : Inport  Port=11
  Fz_rr : Inport  Port=12
  fl : Subsystem
  fr : Subsystem
  rl : Subsystem
  rr : Subsystem
  w_fl : Outport
  w_fr : Outport  Port=2
  w_rl : Outport  Port=3
  w_rr : Outport  Port=4
  wires:
  T_fl/1 -> fl/1(T_fl)
  Fx_fl/1 -> fl/2(Fx_fl)
  Fz_fl/1 -> fl/3(Fz_fl)
  fl/1(w_fl) -> w_fl/1
  fr/1(w_fr) -> w_fr/1
  T_fr/1 -> fr/1(T_fr)
  Fx_fr/1 -> fr/2(Fx_fr)
  Fz_fr/1 -> fr/3(Fz_fr)
  T_rl/1 -> rl/1(T_rl)
  Fx_rl/1 -> rl/2(Fx_rl)
  Fz_rl/1 -> rl/3(Fz_rl)
  rl/1(w_rl) -> w_rl/1
  T_rr/1 -> rr/1(T_rr)
  Fx_rr/1 -> rr/2(Fx_rr)
  Fz_rr/1 -> rr/3(Fz_rr)
  rr/1(w_rr) -> w_rr/1

== system Seven_dof2017a/7DOF_vehicle/alpha_lamda ==
  vx : Inport
  vy : Inport  Port=2
  wz : Inport  Port=3
  delta_fl : Inport  Port=4
  delta_fr : Inport  Port=5
  w_fl : Inport  Port=6
  w_fr : Inport  Port=7
  w_rl : Inport  Port=8
  w_rr : Inport  Port=9
  alpha : Subsystem
  lamda : Subsystem
  lamda_fl : Outport
  lamda_fr : Outport  Port=2
  lamda_rl : Outport  Port=3
  lamda_rr : Outport  Port=4
  alpha_fl : Outport  Port=5
  alpha_fr : Outport  Port=6
  alpha_rl : Outport  Port=7
  alpha_rr : Outport  Port=8
  wires:
  lamda/3(lamda_rl) -> lamda_rl/1
  lamda/4(lamda_rr) -> lamda_rr/1
  lamda/2(lamda_fr) -> lamda_fr/1
  lamda/1(lamda_fl) -> lamda_fl/1
  w_rr/1 -> lamda/9(w_rr)
  w_rl/1 -> lamda/8(w_rl)
  w_fr/1 -> lamda/7(w_fr)
  w_fl/1 -> lamda/6(w_fl)
  delta_fr/1 -> alpha/5(delta_fr), lamda/5(delta_fr)
  delta_fl/1 -> alpha/4(delta_fl), lamda/4(delta_fl)
  wz/1 -> alpha/3(wz), lamda/3(wz)
  vy/1 -> alpha/2(vy), lamda/2(vy)
  vx/1 -> alpha/1(vx), lamda/1(vx)
  alpha/4(alpha_rr) -> alpha_rr/1
  alpha/3(alpha_rl) -> alpha_rl/1
  alpha/2(alpha_fr) -> alpha_fr/1
  alpha/1(alpha_fl) -> alpha_fl/1

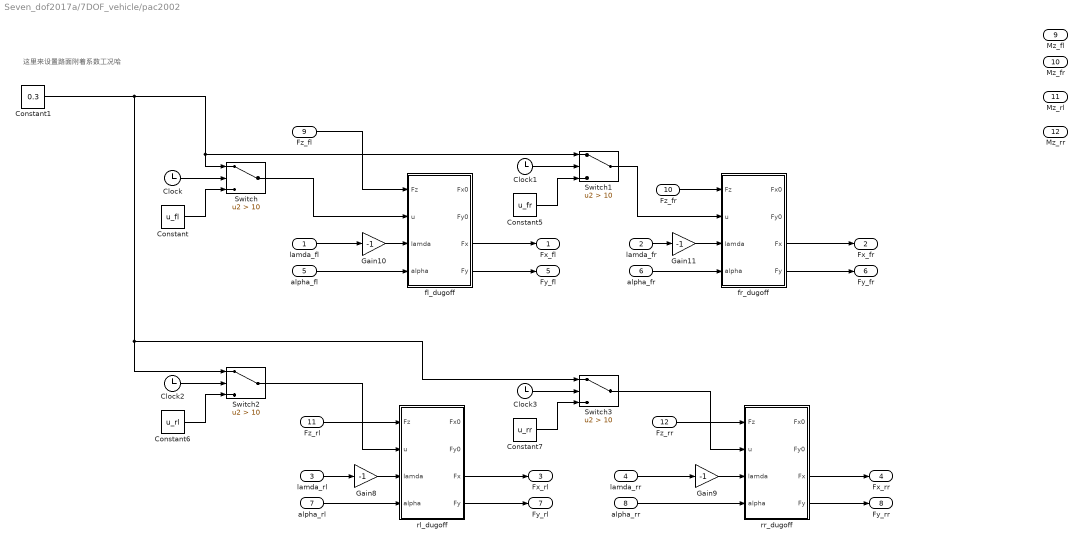
== system Seven_dof2017a/7DOF_vehicle/pac2002 ==
  note: 这里来设置路面附着系数工况哈
  lamda_fl : Inport
  lamda_fr : Inport  Port=2
  lamda_rl : Inport  Port=3
  lamda_rr : Inport  Port=4
  alpha_fl : Inport  Port=5
  alpha_fr : Inport  Port=6
  alpha_rl : Inport  Port=7
  alpha_rr : Inport  Port=8
  Fz_fl : Inport  Port=9
  Fz_fr : Inport  Port=10
  Fz_rl : Inport  Port=11
  Fz_rr : Inport  Port=12
  Clock{,1..3} (4 alike) : Clock
  Constant : Constant  Value=u_fl
  Constant1 : Constant  Value=0.3
  Constant5 : Constant  Value=u_fr
  Constant6 : Constant  Value=u_rl
  Constant7 : Constant  Value=u_rr
  Gain{8..11} (4 alike) : Gain  Gain=-1
  Switch{,1..3} (4 alike) : Switch  Criteria=u2 > Threshold  Threshold=10
  fl_dugoff : MATLAB Function  TreatAsAtomicUnit=on
  fr_dugoff : MATLAB Function  TreatAsAtomicUnit=on
  rl_dugoff : MATLAB Function  TreatAsAtomicUnit=on
  rr_dugoff : MATLAB Function  TreatAsAtomicUnit=on
  Fx_fl : Outport
  Fx_fr : Outport  Port=2
  Fx_rl : Outport  Port=3
  Fx_rr : Outport  Port=4
  Fy_fl : Outport  Port=5
  Fy_fr : Outport  Port=6
  Fy_rl : Outport  Port=7
  Fy_rr : Outport  Port=8
  Mz_fl : Outport  Port=9
  Mz_fr : Outport  Port=10
  Mz_rl : Outport  Port=11
  Mz_rr : Outport  Port=12
  wires:
  alpha_fl/1 -> fl_dugoff/4(alpha)
  Fz_fl/1 -> fl_dugoff/1(Fz)
  Fz_rl/1 -> rl_dugoff/1(Fz)
  alpha_rr/1 -> rr_dugoff/4(alpha)
  Fz_rr/1 -> rr_dugoff/1(Fz)
  Fz_fr/1 -> fr_dugoff/1(Fz)
  fl_dugoff/3(Fx) -> Fx_fl/1
  fl_dugoff/4(Fy) -> Fy_fl/1
  alpha_fr/1 -> fr_dugoff/4(alpha)
  lamda_fr/1 -> Gain11/1
  lamda_rl/1 -> Gain8/1
  lamda_rr/1 -> Gain9/1
  lamda_fl/1 -> Gain10/1
  alpha_rl/1 -> rl_dugoff/4(alpha)
  Gain8/1 -> rl_dugoff/3(lamda)
  Gain9/1 -> rr_dugoff/3(lamda)
  Gain10/1 -> fl_dugoff/3(lamda)
  Gain11/1 -> fr_dugoff/3(lamda)
  fr_dugoff/3(Fx) -> Fx_fr/1
  fr_dugoff/4(Fy) -> Fy_fr/1
  rr_dugoff/3(Fx) -> Fx_rr/1
  rr_dugoff/4(Fy) -> Fy_rr/1
  rl_dugoff/3(Fx) -> Fx_rl/1
  rl_dugoff/4(Fy) -> Fy_rl/1
  Clock/1 -> Switch/2
  Constant/1 -> Switch/3
  Switch/1 -> fl_dugoff/2(u)
  Clock1/1 -> Switch1/2
  Constant5/1 -> Switch1/3
  Switch1/1 -> fr_dugoff/2(u)
  Clock2/1 -> Switch2/2
  Constant6/1 -> Switch2/3
  Switch2/1 -> rl_dugoff/2(u)
  Clock3/1 -> Switch3/2
  Constant7/1 -> Switch3/3
  Switch3/1 -> rr_dugoff/2(u)
  Constant1/1 -> Switch3/1, Switch2/1, Switch1/1, Switch/1

== system Seven_dof2017a/7DOF_vehicle/rad//s_to_rpm ==
  w_fl : Inport
  w_fr : Inport  Port=2
  w_rl : Inport  Port=3
  w_rr : Inport  Port=4
  Gain{,1..3} (4 alike) : Gain  Gain=30/pi
  n_fl : Outport
  n_fr : Outport  Port=2
  n_rl : Outport  Port=3
  n_rr : Outport  Port=4
  tag scope: w_fl=global, w_fr=global, w_rl=global, w_rr=global
  wires:
  Gain3/1 -> n_rr/1
  Gain1/1 -> n_fr/1
  Gain2/1 -> n_rl/1
  w_rl/1 -> [w_rl], Gain2/1
  Gain/1 -> n_fl/1
  w_fl/1 -> [w_fl], Gain/1
  w_fr/1 -> [w_fr], Gain1/1
  w_rr/1 -> [w_rr], Gain3/1

== system Seven_dof2017a/Tyer/Fz ==
  ax : Inport
  ay : Inport  Port=2
  Add : Sum  Inputs=+--
  Add1 : Sum  Inputs=+-+
  Add2 : Sum  Inputs=++-
  Add3 : Sum  Inputs=+++
  Constant : Constant  Value=mw*g+mb*g*Lr/2/L
  Constant1 : Constant  Value=mw*g+mb*g*Lr/2/L
  Constant2 : Constant  Value=mw*g+mb*g*Lf/2/L
  Constant3 : Constant  Value=mw*g+mb*g*Lf/2/L
  Gain : Gain  Gain=mb*hg/2/L
  Gain1 : Gain  Gain=mb*hg/2/Bf
  Fz_fl : Outport
  Fz_fr : Outport  Port=2
  Fz_rl : Outport  Port=3
  Fz_rr : Outport  Port=4
  wires:
  Constant1/1 -> Add1/1
  Constant2/1 -> Add2/1
  Constant/1 -> Add/1
  Gain/1 -> Add3/2, Add2/2, Add1/2, Add/2
  Gain1/1 -> Add3/3, Add2/3, Add1/3, Add/3
  Constant3/1 -> Add3/1
  ay/1 -> Gain1/1
  ax/1 -> Gain/1
  Add3/1 -> Fz_rr/1
  Add2/1 -> Fz_rl/1
  Add1/1 -> Fz_fr/1
  Add/1 -> Fz_fl/1

== system Seven_dof2017a/Tyer/alpha_lamda ==
  vx : Inport
  vy : Inport  Port=2
  wz : Inport  Port=3
  delta_fl : Inport  Port=4
  delta_fr : Inport  Port=5
  w_fl : Inport  Port=6
  w_fr : Inport  Port=7
  w_rl : Inport  Port=8
  w_rr : Inport  Port=9
  alpha : Subsystem
  lamda : Subsystem
  lamda_fl : Outport
  lamda_fr : Outport  Port=2
  lamda_rl : Outport  Port=3
  lamda_rr : Outport  Port=4
  alpha_fl : Outport  Port=5
  alpha_fr : Outport  Port=6
  alpha_rl : Outport  Port=7
  alpha_rr : Outport  Port=8
  wires:
  lamda/3(lamda_rl) -> lamda_rl/1
  lamda/4(lamda_rr) -> lamda_rr/1
  lamda/2(lamda_fr) -> lamda_fr/1
  lamda/1(lamda_fl) -> lamda_fl/1
  w_rr/1 -> lamda/9(w_rr)
  w_rl/1 -> lamda/8(w_rl)
  w_fr/1 -> lamda/7(w_fr)
  w_fl/1 -> lamda/6(w_fl)
  delta_fr/1 -> alpha/5(delta_fr), lamda/5(delta_fr)
  delta_fl/1 -> alpha/4(delta_fl), lamda/4(delta_fl)
  wz/1 -> alpha/3(wz), lamda/3(wz)
  vy/1 -> alpha/2(vy), lamda/2(vy)
  vx/1 -> alpha/1(vx), lamda/1(vx)
  alpha/4(alpha_rr) -> alpha_rr/1
  alpha/3(alpha_rl) -> alpha_rl/1
  alpha/2(alpha_fr) -> alpha_fr/1
  alpha/1(alpha_fl) -> alpha_fl/1

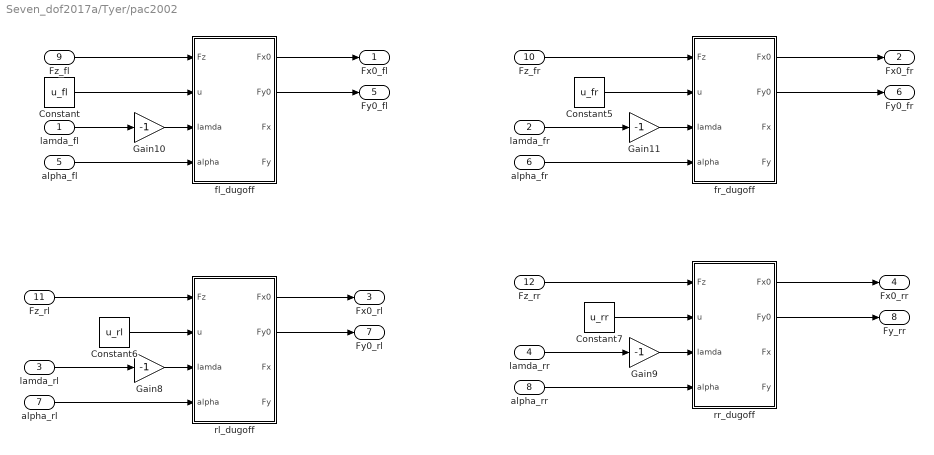
== system Seven_dof2017a/Tyer/pac2002 ==
  lamda_fl : Inport
  lamda_fr : Inport  Port=2
  lamda_rl : Inport  Port=3
  lamda_rr : Inport  Port=4
  alpha_fl : Inport  Port=5
  alpha_fr : Inport  Port=6
  alpha_rl : Inport  Port=7
  alpha_rr : Inport  Port=8
  Fz_fl : Inport  Port=9
  Fz_fr : Inport  Port=10
  Fz_rl : Inport  Port=11
  Fz_rr : Inport  Port=12
  Constant : Constant  Value=u_fl
  Constant5 : Constant  Value=u_fr
  Constant6 : Constant  Value=u_rl
  Constant7 : Constant  Value=u_rr
  Gain{8..11} (4 alike) : Gain  Gain=-1
  fl_dugoff : MATLAB Function  TreatAsAtomicUnit=on
  fr_dugoff : MATLAB Function  TreatAsAtomicUnit=on
  rl_dugoff : MATLAB Function  TreatAsAtomicUnit=on
  rr_dugoff : MATLAB Function  TreatAsAtomicUnit=on
  Fx0_fl : Outport
  Fx0_fr : Outport  Port=2
  Fx0_rl : Outport  Port=3
  Fx0_rr : Outport  Port=4
  Fy0_fl : Outport  Port=5
  Fy0_fr : Outport  Port=6
  Fy0_rl : Outport  Port=7
  Fy_rr : Outport  Port=8
  wires:
  alpha_fl/1 -> fl_dugoff/4(alpha)
  Fz_fl/1 -> fl_dugoff/1(Fz)
  Fz_rl/1 -> rl_dugoff/1(Fz)
  alpha_rr/1 -> rr_dugoff/4(alpha)
  Fz_rr/1 -> rr_dugoff/1(Fz)
  Constant/1 -> fl_dugoff/2(u)
  Fz_fr/1 -> fr_dugoff/1(Fz)
  Constant5/1 -> fr_dugoff/2(u)
  alpha_fr/1 -> fr_dugoff/4(alpha)
  Constant6/1 -> rl_dugoff/2(u)
  Constant7/1 -> rr_dugoff/2(u)
  lamda_fr/1 -> Gain11/1
  lamda_rl/1 -> Gain8/1
  lamda_rr/1 -> Gain9/1
  lamda_fl/1 -> Gain10/1
  fl_dugoff/1(Fx0) -> Fx0_fl/1
  rl_dugoff/1(Fx0) -> Fx0_rl/1
  fl_dugoff/2(Fy0) -> Fy0_fl/1
  fr_dugoff/2(Fy0) -> Fy0_fr/1
  rl_dugoff/2(Fy0) -> Fy0_rl/1
  rr_dugoff/2(Fy0) -> Fy_rr/1
  rr_dugoff/1(Fx0) -> Fx0_rr/1
  alpha_rl/1 -> rl_dugoff/4(alpha)
  Gain8/1 -> rl_dugoff/3(lamda)
  Gain9/1 -> rr_dugoff/3(lamda)
  Gain10/1 -> fl_dugoff/3(lamda)
  Gain11/1 -> fr_dugoff/3(lamda)
  fr_dugoff/1(Fx0) -> Fx0_fr/1

== system Seven_dof2017a/7DOF_vehicle/Body/global system transform ==
  vx : Inport
  vy : Inport  Port=2
  wz : Inport  Port=3
  Add : Sum  Inputs=|+-
  Add1 : Sum  Inputs=|++
  Integrator10 : Integrator
  Integrator8 : Integrator
  Integrator9 : Integrator
  Trigonometric Function1 : Trigonometry
  Trigonometric Function2 : Trigonometry  Operator=cos
  vx*cosr : Product
  vx*sinr : Product
  vy*cosr : Product
  vy*sinr : Product
  x : Outport
  y : Outport  Port=2
  wires:
  vy*cosr/1 -> Add1/2
  Add1/1 -> Integrator9/1
  vx*sinr/1 -> Add1/1
  vx*cosr/1 -> Add/1
  Trigonometric Function1/1 -> vy*sinr/2, vx*sinr/2
  Integrator8/1 -> Trigonometric Function1/1, Trigonometric Function2/1  "r"
  Integrator10/1 -> x/1
  Integrator9/1 -> y/1
  vy/1 -> vy*cosr/1, vy*sinr/1
  wz/1 -> Integrator8/1
  vx/1 -> vx*cosr/1, vx*sinr/1
  vy*sinr/1 -> Add/2
  Trigonometric Function2/1 -> vx*cosr/2, vy*cosr/2
  Add/1 -> Integrator10/1

== system Seven_dof2017a/7DOF_vehicle/Wheel/fl ==
  T_fl : Inport
  Fx_fl : Inport  Port=2
  Fz_fl : Inport  Port=3
  Add : Sum  Inputs=+--
  Constant : Constant  Value=I_tire
  Divide : Product  Inputs=*/
  Gain : Gain  Gain=r
  Gain1 : Gain  Gain=r*f
  Integrator : Integrator  InitialCondition=w0
  w_fl : Outport
  wires:
  Gain/1 -> Add/2
  Fx_fl/1 -> Gain/1
  Fz_fl/1 -> Gain1/1
  T_fl/1 -> Add/1
  Gain1/1 -> Add/3
  Add/1 -> Divide/1
  Constant/1 -> Divide/2
  Divide/1 -> Integrator/1  "dot_w"
  Integrator/1 -> w_fl/1

== system Seven_dof2017a/7DOF_vehicle/Wheel/fr ==
  T_fr : Inport
  Fx_fr : Inport  Port=2
  Fz_fr : Inport  Port=3
  Add : Sum  Inputs=+--
  Constant : Constant  Value=I_tire
  Divide : Product  Inputs=*/
  Gain : Gain  Gain=r
  Gain1 : Gain  Gain=r*f
  Integrator : Integrator  InitialCondition=w0
  w_fr : Outport
  wires:
  Gain1/1 -> Add/3
  Integrator/1 -> w_fr/1
  Divide/1 -> Integrator/1  "dot_w"
  Constant/1 -> Divide/2
  Add/1 -> Divide/1
  Gain/1 -> Add/2
  T_fr/1 -> Add/1
  Fz_fr/1 -> Gain1/1
  Fx_fr/1 -> Gain/1

== system Seven_dof2017a/7DOF_vehicle/Wheel/rl ==
  T_rl : Inport
  Fx_rl : Inport  Port=2
  Fz_rl : Inport  Port=3
  Add : Sum  Inputs=+--
  Constant : Constant  Value=I_tire
  Divide : Product  Inputs=*/
  Gain : Gain  Gain=r
  Gain1 : Gain  Gain=r*f
  Integrator : Integrator  InitialCondition=w0
  w_rl : Outport
  wires:
  Gain1/1 -> Add/3
  Integrator/1 -> w_rl/1
  Divide/1 -> Integrator/1  "dot_w"
  Constant/1 -> Divide/2
  Add/1 -> Divide/1
  Gain/1 -> Add/2
  T_rl/1 -> Add/1
  Fz_rl/1 -> Gain1/1
  Fx_rl/1 -> Gain/1

== system Seven_dof2017a/7DOF_vehicle/Wheel/rr ==
  T_rr : Inport
  Fx_rr : Inport  Port=2
  Fz_rr : Inport  Port=3
  Add : Sum  Inputs=+--
  Constant : Constant  Value=I_tire
  Divide : Product  Inputs=*/
  Gain : Gain  Gain=r
  Gain1 : Gain  Gain=r*f
  Integrator : Integrator  InitialCondition=w0
  w_rr : Outport
  wires:
  Gain1/1 -> Add/3
  Fx_rr/1 -> Gain/1
  Fz_rr/1 -> Gain1/1
  T_rr/1 -> Add/1
  Gain/1 -> Add/2
  Add/1 -> Divide/1
  Constant/1 -> Divide/2
  Divide/1 -> Integrator/1  "dot_w"
  Integrator/1 -> w_rr/1

== system Seven_dof2017a/7DOF_vehicle/alpha_lamda/alpha ==
  vx : Inport
  vy : Inport  Port=2
  wz : Inport  Port=3
  delta_fl : Inport  Port=4
  delta_fr : Inport  Port=5
  Gain{,1..3} (4 alike) : Gain  Gain=-1
  fl : Subsystem
  fr : Subsystem
  rl : Subsystem
  rr : Subsystem
  alpha_fl : Outport
  alpha_fr : Outport  Port=2
  alpha_rl : Outport  Port=3
  alpha_rr : Outport  Port=4
  wires:
  delta_fr/1 -> fr/4(delta_fr)
  delta_fl/1 -> fl/4(delta_fl)
  vy/1 -> rl/2(vy), fl/2(vy), fr/2(vy), rr/2(vy)
  vx/1 -> rl/1(vx), fl/1(vx), fr/1(vx), rr/1(vx)
  wz/1 -> rl/3(wz), fr/3(wz), rr/3(wz), fl/3(wz)
  fl/1(alpha_fl) -> Gain/1
  Gain/1 -> alpha_fl/1
  rl/1(alpha_rl) -> Gain1/1
  Gain1/1 -> alpha_rl/1
  fr/1(alpha_fr) -> Gain2/1
  Gain2/1 -> alpha_fr/1
  rr/1(alpha_rr) -> Gain3/1
  Gain3/1 -> alpha_rr/1

== system Seven_dof2017a/7DOF_vehicle/alpha_lamda/lamda ==
  vx : Inport
  vy : Inport  Port=2
  wz : Inport  Port=3
  delta_fl : Inport  Port=4
  delta_fr : Inport  Port=5
  w_fl : Inport  Port=6
  w_fr : Inport  Port=7
  w_rl : Inport  Port=8
  w_rr : Inport  Port=9
  fl : Subsystem
  fr : Subsystem
  rl : Subsystem
  rr : Subsystem
  lamda_fl : Outport
  lamda_fr : Outport  Port=2
  lamda_rl : Outport  Port=3
  lamda_rr : Outport  Port=4
  wires:
  fr/1(lamda_fr) -> lamda_fr/1
  rr/1(lamda_rr) -> lamda_rr/1
  w_rl/1 -> rl/1(w_rl)
  w_rr/1 -> rr/1(w_rr)
  w_fr/1 -> fr/1(w_fr)
  delta_fr/1 -> fr/5(delta_fr)
  delta_fl/1 -> fl/5(delta_fl)
  vy/1 -> fl/4(vy), fr/4(vy)
  vx/1 -> fl/3(vx), fr/3(vx), rr/3(vx), rl/3(vx)
  wz/1 -> fl/2(wz), fr/2(wz), rr/2(wz), rl/2(wz)
  w_fl/1 -> fl/1(w_fl)
  rl/1(lamda_rl) -> lamda_rl/1
  fl/1(lamda_fl) -> lamda_fl/1

== system Seven_dof2017a/Tyer/alpha_lamda/alpha ==
  vx : Inport
  vy : Inport  Port=2
  wz : Inport  Port=3
  delta_fl : Inport  Port=4
  delta_fr : Inport  Port=5
  Gain{,1..3} (4 alike) : Gain  Gain=-1
  fl : Subsystem
  fr : Subsystem
  rl : Subsystem
  rr : Subsystem
  alpha_fl : Outport
  alpha_fr : Outport  Port=2
  alpha_rl : Outport  Port=3
  alpha_rr : Outport  Port=4
  wires:
  delta_fr/1 -> fr/4(delta_fr)
  delta_fl/1 -> fl/4(delta_fl)
  vy/1 -> rl/2(vy), fl/2(vy), fr/2(vy), rr/2(vy)
  vx/1 -> rl/1(vx), fl/1(vx), fr/1(vx), rr/1(vx)
  wz/1 -> rl/3(wz), fr/3(wz), rr/3(wz), fl/3(wz)
  fl/1(alpha_fl) -> Gain/1
  Gain/1 -> alpha_fl/1
  rl/1(alpha_rl) -> Gain1/1
  Gain1/1 -> alpha_rl/1
  fr/1(alpha_fr) -> Gain2/1
  Gain2/1 -> alpha_fr/1
  rr/1(alpha_rr) -> Gain3/1
  Gain3/1 -> alpha_rr/1

== system Seven_dof2017a/Tyer/alpha_lamda/lamda ==
  vx : Inport
  vy : Inport  Port=2
  wz : Inport  Port=3
  delta_fl : Inport  Port=4
  delta_fr : Inport  Port=5
  w_fl : Inport  Port=6
  w_fr : Inport  Port=7
  w_rl : Inport  Port=8
  w_rr : Inport  Port=9
  fl : Subsystem
  fr : Subsystem
  rl : Subsystem
  rr : Subsystem
  lamda_fl : Outport
  lamda_fr : Outport  Port=2
  lamda_rl : Outport  Port=3
  lamda_rr : Outport  Port=4
  wires:
  fr/1(lamda_fr) -> lamda_fr/1
  rr/1(lamda_rr) -> lamda_rr/1
  w_rl/1 -> rl/1(w_rl)
  w_rr/1 -> rr/1(w_rr)
  w_fr/1 -> fr/1(w_fr)
  delta_fr/1 -> fr/5(delta_fr)
  delta_fl/1 -> fl/5(delta_fl)
  vy/1 -> fl/4(vy), fr/4(vy)
  vx/1 -> fl/3(vx), fr/3(vx), rr/3(vx), rl/3(vx)
  wz/1 -> fl/2(wz), fr/2(wz), rr/2(wz), rl/2(wz)
  w_fl/1 -> fl/1(w_fl)
  rl/1(lamda_rl) -> lamda_rl/1
  fl/1(lamda_fl) -> lamda_fl/1

== system Seven_dof2017a/7DOF_vehicle/alpha_lamda/alpha/fl ==
  vx : Inport
  vy : Inport  Port=2
  wz : Inport  Port=3
  delta_fl : Inport  Port=4
  Add2 : Sum
  Add3 : Sum  Inputs=+-
  Add4 : Sum  Inputs=-+
  Divide : Product  Inputs=/*
  Gain3 : Gain  Gain=Lf
  Gain4 : Gain  Gain=0.5*Bf
  Trigonometric Function : Trigonometry  Operator=atan
  alpha_fl : Outport
  wires:
  wz/1 -> Gain3/1, Gain4/1
  Add4/1 -> alpha_fl/1
  vy/1 -> Add2/1
  delta_fl/1 -> Add4/2
  vx/1 -> Add3/1
  Trigonometric Function/1 -> Add4/1
  Divide/1 -> Trigonometric Function/1
  Add3/1 -> Divide/1
  Add2/1 -> Divide/2
  Gain4/1 -> Add3/2
  Gain3/1 -> Add2/2

== system Seven_dof2017a/7DOF_vehicle/alpha_lamda/alpha/fr ==
  vx : Inport
  vy : Inport  Port=2
  wz : Inport  Port=3
  delta_fr : Inport  Port=4
  Add2 : Sum
  Add3 : Sum
  Add4 : Sum  Inputs=-+
  Divide : Product  Inputs=/*
  Gain3 : Gain  Gain=Lf
  Gain4 : Gain  Gain=0.5*Bf
  Trigonometric Function : Trigonometry  Operator=atan
  alpha_fr : Outport
  wires:
  Gain3/1 -> Add2/2
  Add2/1 -> Divide/2
  Add3/1 -> Divide/1
  Divide/1 -> Trigonometric Function/1
  Trigonometric Function/1 -> Add4/1
  vx/1 -> Add3/1
  delta_fr/1 -> Add4/2
  vy/1 -> Add2/1
  Add4/1 -> alpha_fr/1
  wz/1 -> Gain4/1, Gain3/1
  Gain4/1 -> Add3/2

== system Seven_dof2017a/7DOF_vehicle/alpha_lamda/alpha/rl ==
  vx : Inport
  vy : Inport  Port=2
  wz : Inport  Port=3
  Add2 : Sum  Inputs=+-
  Add3 : Sum  Inputs=+-
  Divide : Product  Inputs=/*
  Gain1 : Gain  Gain=-1
  Gain3 : Gain  Gain=Lr
  Gain4 : Gain  Gain=0.5*Br
  Trigonometric Function : Trigonometry  Operator=atan
  alpha_rl : Outport
  wires:
  Gain3/1 -> Add2/2
  Add2/1 -> Divide/2
  Add3/1 -> Divide/1
  Divide/1 -> Trigonometric Function/1
  vx/1 -> Add3/1
  vy/1 -> Add2/1
  wz/1 -> Gain4/1, Gain3/1
  Trigonometric Function/1 -> Gain1/1
  Gain4/1 -> Add3/2
  Gain1/1 -> alpha_rl/1

== system Seven_dof2017a/7DOF_vehicle/alpha_lamda/alpha/rr ==
  vx : Inport
  vy : Inport  Port=2
  wz : Inport  Port=3
  Add2 : Sum  Inputs=+-
  Add3 : Sum
  Divide : Product  Inputs=/*
  Gain2 : Gain  Gain=-1
  Gain3 : Gain  Gain=Lr
  Gain4 : Gain  Gain=0.5*Br
  Trigonometric Function : Trigonometry  Operator=atan
  alpha_rr : Outport
  wires:
  Trigonometric Function/1 -> Gain2/1
  wz/1 -> Gain3/1, Gain4/1
  vy/1 -> Add2/1
  vx/1 -> Add3/1
  Divide/1 -> Trigonometric Function/1
  Add3/1 -> Divide/1
  Add2/1 -> Divide/2
  Gain3/1 -> Add2/2
  Gain4/1 -> Add3/2
  Gain2/1 -> alpha_rr/1

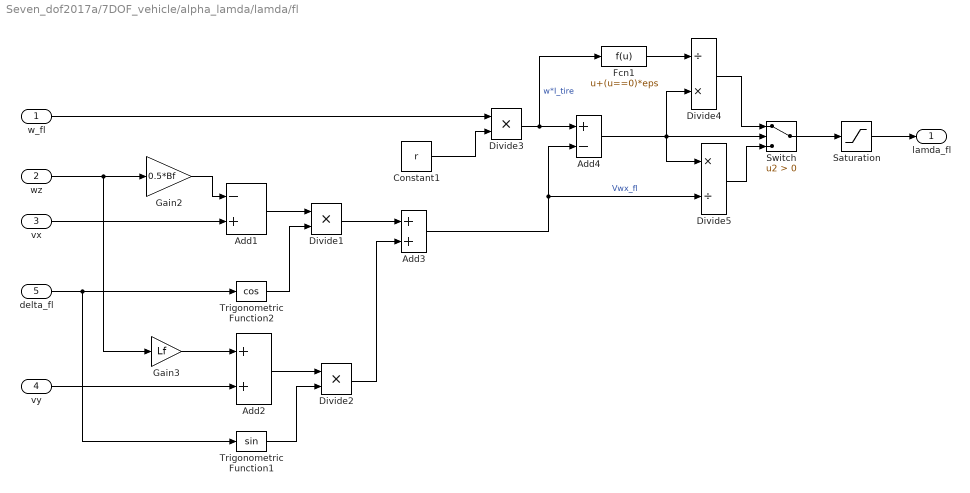
== system Seven_dof2017a/7DOF_vehicle/alpha_lamda/lamda/fl ==
  w_fl : Inport
  wz : Inport  Port=2
  vx : Inport  Port=3
  vy : Inport  Port=4
  delta_fl : Inport  Port=5
  Add1 : Sum  Inputs=-+
  Add2 : Sum
  Add3 : Sum
  Add4 : Sum  Inputs=+-
  Constant1 : Constant  Value=r
  Divide1 : Product  Inputs=**
  Divide2 : Product  Inputs=**
  Divide3 : Product  Inputs=**
  Divide4 : Product  Inputs=/*
  Divide5 : Product  Inputs=*/
  Fcn1 : Fcn  Expr=u+(u==0)*eps
  Gain2 : Gain  Gain=0.5*Bf
  Gain3 : Gain  Gain=Lf
  Saturation : Saturate  UpperLimit=1  LowerLimit=-1
  Switch : Switch  Criteria=u2 > Threshold
  Trigonometric Function1 : Trigonometry
  Trigonometric Function2 : Trigonometry  Operator=cos
  lamda_fl : Outport
  wires:
  Switch/1 -> Saturation/1
  Add3/1 -> Add4/2, Divide5/2  "Vwx_fl"
  Add4/1 -> Switch/2, Divide4/2, Divide5/1
  Divide4/1 -> Switch/1
  Divide5/1 -> Switch/3
  Fcn1/1 -> Divide4/1
  vx/1 -> Add1/2
  Gain2/1 -> Add1/1
  wz/1 -> Gain3/1, Gain2/1
  Add1/1 -> Divide1/1
  delta_fl/1 -> Trigonometric Function2/1, Trigonometric Function1/1
  Trigonometric Function2/1 -> Divide1/2
  vy/1 -> Add2/2
  Gain3/1 -> Add2/1
  Add2/1 -> Divide2/1
  Trigonometric Function1/1 -> Divide2/2
  Divide1/1 -> Add3/1
  Divide2/1 -> Add3/2
  w_fl/1 -> Divide3/1
  Constant1/1 -> Divide3/2
  Divide3/1 -> Add4/1, Fcn1/1  "w*I_tire"
  Saturation/1 -> lamda_fl/1

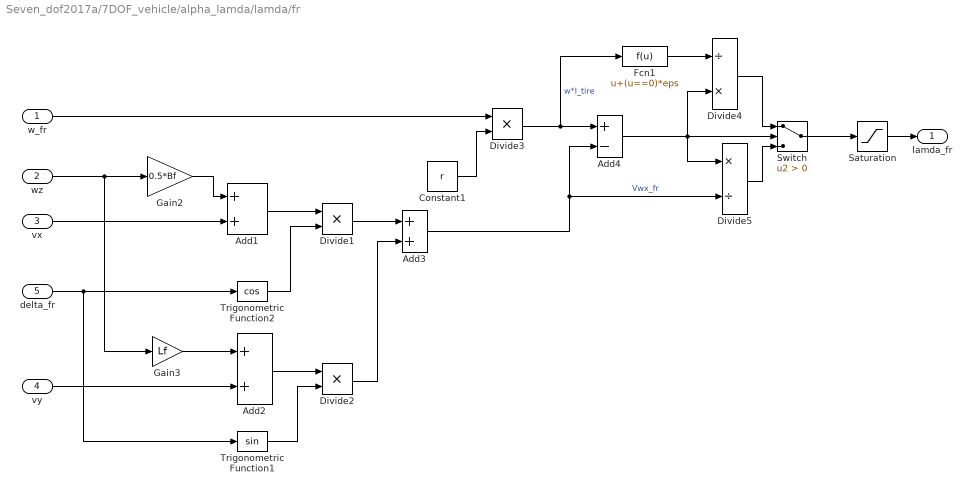
== system Seven_dof2017a/7DOF_vehicle/alpha_lamda/lamda/fr ==
  w_fr : Inport
  wz : Inport  Port=2
  vx : Inport  Port=3
  vy : Inport  Port=4
  delta_fr : Inport  Port=5
  Add1 : Sum
  Add2 : Sum
  Add3 : Sum
  Add4 : Sum  Inputs=+-
  Constant1 : Constant  Value=r
  Divide1 : Product  Inputs=**
  Divide2 : Product  Inputs=**
  Divide3 : Product  Inputs=**
  Divide4 : Product  Inputs=/*
  Divide5 : Product  Inputs=*/
  Fcn1 : Fcn  Expr=u+(u==0)*eps
  Gain2 : Gain  Gain=0.5*Bf
  Gain3 : Gain  Gain=Lf
  Saturation : Saturate  UpperLimit=1  LowerLimit=-1
  Switch : Switch  Criteria=u2 > Threshold
  Trigonometric Function1 : Trigonometry
  Trigonometric Function2 : Trigonometry  Operator=cos
  lamda_fr : Outport
  wires:
  Saturation/1 -> lamda_fr/1
  vx/1 -> Add1/2
  Gain2/1 -> Add1/1
  wz/1 -> Gain3/1, Gain2/1
  Add1/1 -> Divide1/1
  delta_fr/1 -> Trigonometric Function2/1, Trigonometric Function1/1
  Trigonometric Function2/1 -> Divide1/2
  vy/1 -> Add2/2
  Gain3/1 -> Add2/1
  Add2/1 -> Divide2/1
  Trigonometric Function1/1 -> Divide2/2
  Divide1/1 -> Add3/1
  Divide2/1 -> Add3/2
  w_fr/1 -> Divide3/1
  Constant1/1 -> Divide3/2
  Divide3/1 -> Fcn1/1, Add4/1  "w*I_tire"
  Fcn1/1 -> Divide4/1
  Divide5/1 -> Switch/3
  Divide4/1 -> Switch/1
  Add4/1 -> Divide5/1, Divide4/2, Switch/2
  Add3/1 -> Divide5/2, Add4/2  "Vwx_fr"
  Switch/1 -> Saturation/1

== system Seven_dof2017a/7DOF_vehicle/alpha_lamda/lamda/rl ==
  w_rl : Inport
  wz : Inport  Port=2
  vx : Inport  Port=3
  Add1 : Sum  Inputs=-+
  Add4 : Sum  Inputs=+-
  Constant1 : Constant  Value=r
  Divide3 : Product  Inputs=**
  Divide4 : Product  Inputs=/*
  Divide5 : Product  Inputs=*/
  Fcn1 : Fcn  Expr=u+(u==0)*eps
  Gain2 : Gain  Gain=0.5*Br
  Saturation : Saturate  UpperLimit=1  LowerLimit=-1
  Switch : Switch  Criteria=u2 > Threshold
  lamda_rl : Outport
  wires:
  Saturation/1 -> lamda_rl/1
  vx/1 -> Add1/2
  Gain2/1 -> Add1/1
  wz/1 -> Gain2/1
  w_rl/1 -> Divide3/1
  Constant1/1 -> Divide3/2
  Divide3/1 -> Fcn1/1, Add4/1  "w*I_tire"
  Fcn1/1 -> Divide4/1
  Divide5/1 -> Switch/3
  Divide4/1 -> Switch/1
  Add4/1 -> Divide5/1, Divide4/2, Switch/2
  Add1/1 -> Divide5/2, Add4/2
  Switch/1 -> Saturation/1

== system Seven_dof2017a/7DOF_vehicle/alpha_lamda/lamda/rr ==
  w_rr : Inport
  wz : Inport  Port=2
  vx : Inport  Port=3
  Add1 : Sum
  Add4 : Sum  Inputs=+-
  Constant1 : Constant  Value=r
  Divide3 : Product  Inputs=**
  Divide4 : Product  Inputs=/*
  Divide5 : Product  Inputs=*/
  Fcn1 : Fcn  Expr=u+(u==0)*eps
  Gain2 : Gain  Gain=0.5*Br
  Saturation : Saturate  UpperLimit=1  LowerLimit=-1
  Switch : Switch  Criteria=u2 > Threshold
  lamda_rr : Outport
  wires:
  Saturation/1 -> lamda_rr/1
  Switch/1 -> Saturation/1
  Constant1/1 -> Divide3/2
  w_rr/1 -> Divide3/1
  wz/1 -> Gain2/1
  Gain2/1 -> Add1/1
  vx/1 -> Add1/2
  Divide3/1 -> Fcn1/1, Add4/1  "w*I_tire"
  Fcn1/1 -> Divide4/1
  Divide5/1 -> Switch/3
  Divide4/1 -> Switch/1
  Add4/1 -> Divide5/1, Divide4/2, Switch/2
  Add1/1 -> Divide5/2, Add4/2  "Vwx_rr"

== system Seven_dof2017a/Tyer/alpha_lamda/alpha/fl ==
  vx : Inport
  vy : Inport  Port=2
  wz : Inport  Port=3
  delta_fl : Inport  Port=4
  Add2 : Sum
  Add3 : Sum  Inputs=+-
  Add4 : Sum  Inputs=-+
  Divide : Product  Inputs=/*
  Gain3 : Gain  Gain=Lf
  Gain4 : Gain  Gain=0.5*Bf
  Trigonometric Function : Trigonometry  Operator=atan
  alpha_fl : Outport
  wires:
  wz/1 -> Gain3/1, Gain4/1
  Add4/1 -> alpha_fl/1
  vy/1 -> Add2/1
  delta_fl/1 -> Add4/2
  vx/1 -> Add3/1
  Trigonometric Function/1 -> Add4/1
  Divide/1 -> Trigonometric Function/1
  Add3/1 -> Divide/1
  Add2/1 -> Divide/2
  Gain4/1 -> Add3/2
  Gain3/1 -> Add2/2

== system Seven_dof2017a/Tyer/alpha_lamda/alpha/fr ==
  vx : Inport
  vy : Inport  Port=2
  wz : Inport  Port=3
  delta_fr : Inport  Port=4
  Add2 : Sum
  Add3 : Sum
  Add4 : Sum  Inputs=-+
  Divide : Product  Inputs=/*
  Gain3 : Gain  Gain=Lf
  Gain4 : Gain  Gain=0.5*Bf
  Trigonometric Function : Trigonometry  Operator=atan
  alpha_fr : Outport
  wires:
  Gain3/1 -> Add2/2
  Add2/1 -> Divide/2
  Add3/1 -> Divide/1
  Divide/1 -> Trigonometric Function/1
  Trigonometric Function/1 -> Add4/1
  vx/1 -> Add3/1
  delta_fr/1 -> Add4/2
  vy/1 -> Add2/1
  Add4/1 -> alpha_fr/1
  wz/1 -> Gain4/1, Gain3/1
  Gain4/1 -> Add3/2

== system Seven_dof2017a/Tyer/alpha_lamda/alpha/rl ==
  vx : Inport
  vy : Inport  Port=2
  wz : Inport  Port=3
  Add2 : Sum  Inputs=+-
  Add3 : Sum  Inputs=+-
  Divide : Product  Inputs=/*
  Gain1 : Gain  Gain=-1
  Gain3 : Gain  Gain=Lr
  Gain4 : Gain  Gain=0.5*Br
  Trigonometric Function : Trigonometry  Operator=atan
  alpha_rl : Outport
  wires:
  Gain3/1 -> Add2/2
  Add2/1 -> Divide/2
  Add3/1 -> Divide/1
  Divide/1 -> Trigonometric Function/1
  vx/1 -> Add3/1
  vy/1 -> Add2/1
  wz/1 -> Gain4/1, Gain3/1
  Trigonometric Function/1 -> Gain1/1
  Gain4/1 -> Add3/2
  Gain1/1 -> alpha_rl/1

== system Seven_dof2017a/Tyer/alpha_lamda/alpha/rr ==
  vx : Inport
  vy : Inport  Port=2
  wz : Inport  Port=3
  Add2 : Sum  Inputs=+-
  Add3 : Sum
  Divide : Product  Inputs=/*
  Gain2 : Gain  Gain=-1
  Gain3 : Gain  Gain=Lr
  Gain4 : Gain  Gain=0.5*Br
  Trigonometric Function : Trigonometry  Operator=atan
  alpha_rr : Outport
  wires:
  Trigonometric Function/1 -> Gain2/1
  wz/1 -> Gain3/1, Gain4/1
  vy/1 -> Add2/1
  vx/1 -> Add3/1
  Divide/1 -> Trigonometric Function/1
  Add3/1 -> Divide/1
  Add2/1 -> Divide/2
  Gain3/1 -> Add2/2
  Gain4/1 -> Add3/2
  Gain2/1 -> alpha_rr/1

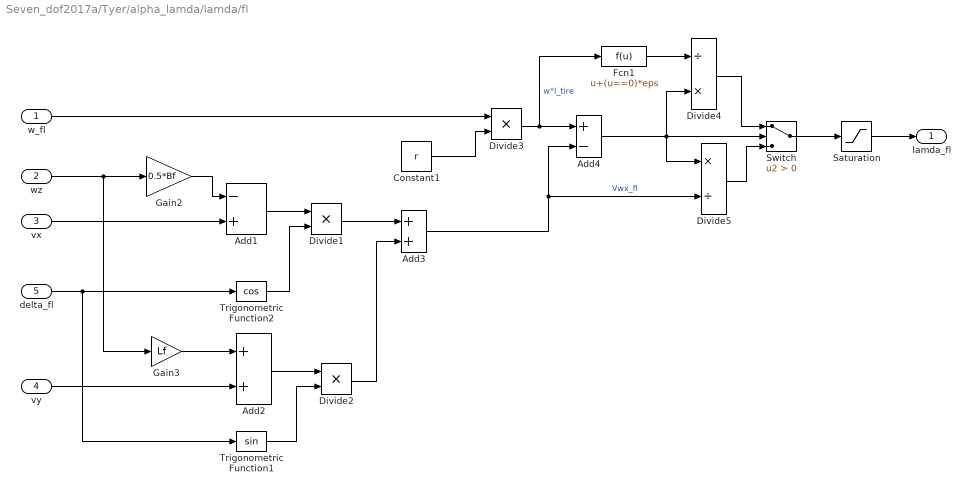
== system Seven_dof2017a/Tyer/alpha_lamda/lamda/fl ==
  w_fl : Inport
  wz : Inport  Port=2
  vx : Inport  Port=3
  vy : Inport  Port=4
  delta_fl : Inport  Port=5
  Add1 : Sum  Inputs=-+
  Add2 : Sum
  Add3 : Sum
  Add4 : Sum  Inputs=+-
  Constant1 : Constant  Value=r
  Divide1 : Product  Inputs=**
  Divide2 : Product  Inputs=**
  Divide3 : Product  Inputs=**
  Divide4 : Product  Inputs=/*
  Divide5 : Product  Inputs=*/
  Fcn1 : Fcn  Expr=u+(u==0)*eps
  Gain2 : Gain  Gain=0.5*Bf
  Gain3 : Gain  Gain=Lf
  Saturation : Saturate  UpperLimit=1  LowerLimit=-1
  Switch : Switch  Criteria=u2 > Threshold
  Trigonometric Function1 : Trigonometry
  Trigonometric Function2 : Trigonometry  Operator=cos
  lamda_fl : Outport
  wires:
  Switch/1 -> Saturation/1
  Add3/1 -> Add4/2, Divide5/2  "Vwx_fl"
  Add4/1 -> Switch/2, Divide4/2, Divide5/1
  Divide4/1 -> Switch/1
  Divide5/1 -> Switch/3
  Fcn1/1 -> Divide4/1
  vx/1 -> Add1/2
  Gain2/1 -> Add1/1
  wz/1 -> Gain3/1, Gain2/1
  Add1/1 -> Divide1/1
  delta_fl/1 -> Trigonometric Function2/1, Trigonometric Function1/1
  Trigonometric Function2/1 -> Divide1/2
  vy/1 -> Add2/2
  Gain3/1 -> Add2/1
  Add2/1 -> Divide2/1
  Trigonometric Function1/1 -> Divide2/2
  Divide1/1 -> Add3/1
  Divide2/1 -> Add3/2
  w_fl/1 -> Divide3/1
  Constant1/1 -> Divide3/2
  Divide3/1 -> Add4/1, Fcn1/1  "w*I_tire"
  Saturation/1 -> lamda_fl/1
